simulink library "MMC_Lib"  (R2023b)
settings: Solver=VariableStepAuto  StartTime=0.0  StopTime=10.0  RelTol=1e-3
undefined symbols (not defined in the file): C_PM, D_R, D_Rs, DiscIntNeverNeededParam, Discrete, Nb_PM, spsDiodeModel, Ts_Power
libraries: simulink x23, simulink_extras x1, $bdroot x1
settings Model: Creator=rober  LastModifiedBy=rober

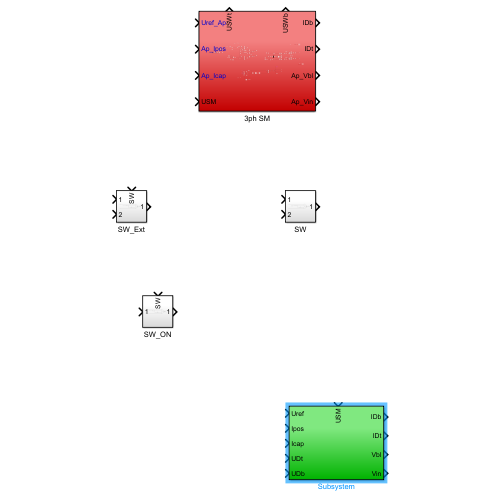
[thumbnail: Simulink's stored preview of the top-level diagram]
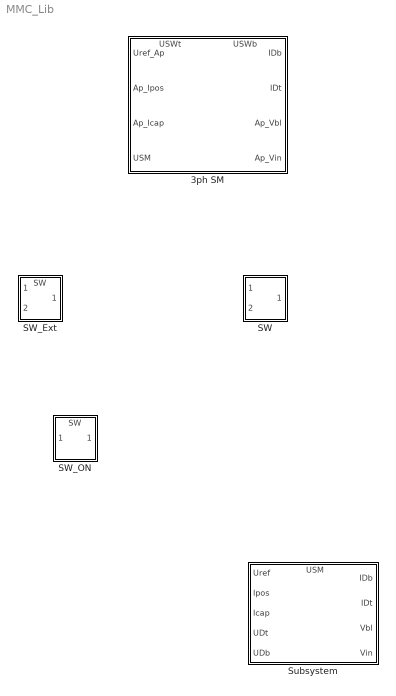
== system MMC_Lib ==
  3ph SM : Subsystem
      settings: PortSchema="{\"entries\":[{\"content\":{\"sides\":[{\"content\":{\"connectorIds\":[\"In1\",\"In2\",\"In3\",\"In4\"]},\"type\":\"ConnectorPlacement.EquallySpacedRectSide\",\"uuid\":\"e8c5836a-6fd4-401e-94d8-c7848e2937c8\"},{\"content\":{\"connectorIds\":[\"Out1\",\"Out2\",\"Out3\",\"Out4\"],\"side\":\"RIGHT\"},\"type\":\"ConnectorPlacement.EquallySpacedRectSide\",\"uuid\":\"9a1f81e7-802a-4d89-b611-499076d5a1a3\"},{\"content\":{\"connectorIds\":[\"Out5\",\"Out6\"],\"side\":\"TOP\"},\"type\":\"ConnectorPlacement.EquallySpacedRectSide\",\"uuid\":\"c5bcecc8-9b4b-4040-ad1a-25d769dc4514\"}]},\"type\":\"ConnectorPlacement.EquallySpacedConnector\",\"uuid\":\"eb5ff5d9-ed1d-4618-9338-8ec7700f9d1e\"}],\"packageUris\":[\"http://schema.mathworks.com/mf0/Connector/R2020b\"],\"version\":\"1.0\"}"
  SW : Subsystem
  SW_Ext : Subsystem
      settings: PortSchema="{\"entries\":[{\"content\":{\"sides\":[{\"content\":{\"connectorIds\":[\"In1\",\"In2\"]},\"type\":\"ConnectorPlacement.EquallySpacedRectSide\",\"uuid\":\"61570b56-e5d0-4812-b143-8fea08408b82\"},{\"content\":{\"connectorIds\":[\"Out1\"],\"side\":\"RIGHT\"},\"type\":\"ConnectorPlacement.EquallySpacedRectSide\",\"uuid\":\"fb1b449d-dcf0-4498-bfcd-c35d1b8d3af1\"},{\"content\":{\"connectorIds\":[\"In3\"],\"side\":\"TOP\"},\"type\":\"ConnectorPlacement.EquallySpacedRectSide\",\"uuid\":\"2091de1c-d6a0-4f6b-9728-c6eb9657220b\"}]},\"type\":\"ConnectorPlacement.EquallySpacedConnector\",\"uuid\":\"fce121a6-5cfd-4a9e-88a9-d62df4eca96b\"}],\"packageUris\":[\"http://schema.mathworks.com/mf0/Connector/R2020b\"],\"version\":\"1.0\"}"
  SW_ON : Subsystem
      settings: PortSchema="{\"entries\":[{\"content\":{\"sides\":[{\"content\":{\"connectorIds\":[\"In1\"]},\"type\":\"ConnectorPlacement.EquallySpacedRectSide\",\"uuid\":\"61570b56-e5d0-4812-b143-8fea08408b82\"},{\"content\":{\"connectorIds\":[\"Out1\"],\"side\":\"RIGHT\"},\"type\":\"ConnectorPlacement.EquallySpacedRectSide\",\"uuid\":\"fb1b449d-dcf0-4498-bfcd-c35d1b8d3af1\"},{\"content\":{\"connectorIds\":[\"In2\"],\"side\":\"TOP\"},\"type\":\"ConnectorPlacement.EquallySpacedRectSide\",\"uuid\":\"2091de1c-d6a0-4f6b-9728-c6eb9657220b\"}]},\"type\":\"ConnectorPlacement.EquallySpacedConnector\",\"uuid\":\"fce121a6-5cfd-4a9e-88a9-d62df4eca96b\"}],\"packageUris\":[\"http://schema.mathworks.com/mf0/Connector/R2020b\"],\"version\":\"1.0\"}"
  Subsystem : Subsystem
      settings: PortSchema="{\"entries\":[{\"content\":{\"sides\":[{\"content\":{\"connectorIds\":[\"In1\",\"In2\",\"In3\",\"In4\",\"In5\"]},\"type\":\"ConnectorPlacement.EquallySpacedRectSide\",\"uuid\":\"b7415a3a-059a-466d-a519-c19f63b714af\"},{\"content\":{\"connectorIds\":[\"Out1\",\"Out2\",\"Out3\",\"Out4\"],\"side\":\"RIGHT\"},\"type\":\"ConnectorPlacement.EquallySpacedRectSide\",\"uuid\":\"984beb61-c57c-4d2a-959b-3a61047ea667\"},{\"content\":{\"connectorIds\":[\"In6\"],\"side\":\"TOP\"},\"type\":\"ConnectorPlacement.EquallySpacedRectSide\",\"uuid\":\"184f05c1-6fe5-4e4c-8e83-c1431acf6740\"}]},\"type\":\"ConnectorPlacement.EquallySpacedConnector\",\"uuid\":\"ac4715c0-a7f3-4877-877b-fb86a389a1b7\"}],\"packageUris\":[\"http://schema.mathworks.com/mf0/Connector/R2020b\"],\"version\":\"1.0\"}"

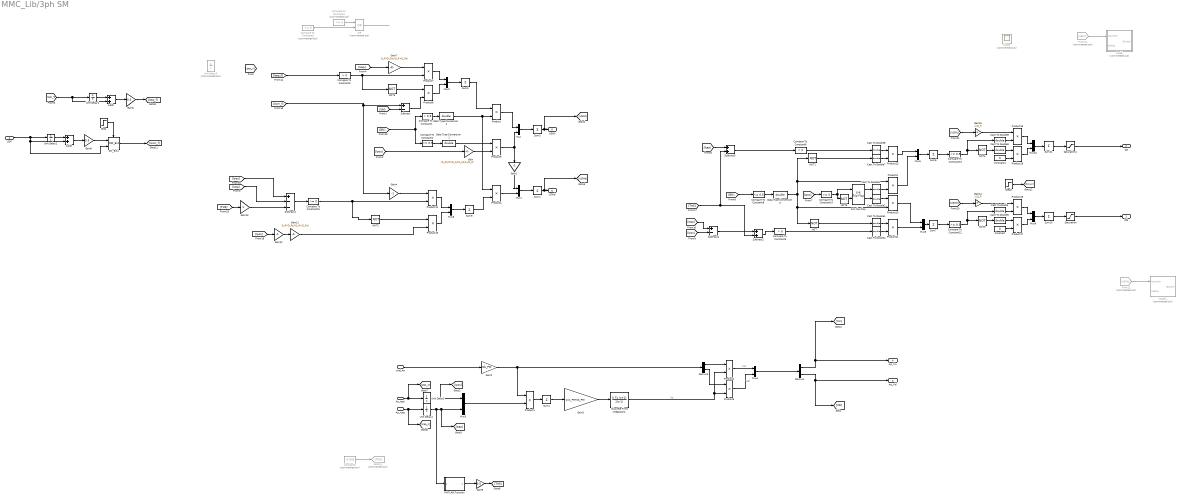
== system MMC_Lib/3ph SM ==
  Uref_Ap : Inport
  Ap_Ipos : Inport  Port=2
  Ap_Icap : Inport  Port=3
  USM : Inport  Port=4
  Add2 : Sum
  Add3 : Sum
  Cast To Double{,1..9} (10 alike) : DataTypeConversion  OutDataTypeStr=double  SaturateOnIntegerOverflow=off  RndMeth=Floor
  Compare To Constant1 : simulink/Logic and Bit Operations/Compare To Constant  relop=>  const=0.5  OutDataTypeStr=boolean
  Compare To Constant10 : simulink/Logic and Bit Operations/Compare To Constant  relop=>=  const=0  OutDataTypeStr=boolean
  Compare To Constant12 : simulink/Logic and Bit Operations/Compare To Constant  relop=>=  const=0.5  OutDataTypeStr=boolean
  Compare To Constant13 : simulink/Logic and Bit Operations/Compare To Constant  relop=>=  const=0.5  OutDataTypeStr=boolean
  Compare To Constant14 : simulink/Logic and Bit Operations/Compare To Constant  relop=>=  const=0  OutDataTypeStr=boolean
  Compare To Constant2 : simulink/Logic and Bit Operations/Compare To Constant  relop=<=  const=0.5  OutDataTypeStr=boolean
  Compare To Constant3 : simulink/Logic and Bit Operations/Compare To Constant  relop=>  const=0  OutDataTypeStr=boolean
  Compare To Constant4 : simulink/Logic and Bit Operations/Compare To Constant  Commented=on  relop=<=  const=0  OutDataTypeStr=boolean
  Compare To Constant5 : simulink/Logic and Bit Operations/Compare To Constant  Commented=on  relop=<=  const=0  OutDataTypeStr=boolean
  Compare To Constant6 : simulink/Logic and Bit Operations/Compare To Constant  relop=>  const=0  OutDataTypeStr=boolean
  Compare To Constant8 : simulink/Logic and Bit Operations/Compare To Constant  relop=<=  const=0.5  OutDataTypeStr=boolean
  Compare To Constant9 : simulink/Logic and Bit Operations/Compare To Constant  relop=>  const=0  OutDataTypeStr=boolean
  Constant : Constant  Value=0
  Constant1 : Constant  Value=0
  Constant2 : Constant  Commented=on  Value=-0.003
  Data Type Conversion1 : DataTypeConversion  OutDataTypeStr=double  SaturateOnIntegerOverflow=off  RndMeth=Floor
  Data Type Conversion2 : DataTypeConversion  OutDataTypeStr=double  SaturateOnIntegerOverflow=off  RndMeth=Floor
  Data Type Conversion3 : DataTypeConversion  OutDataTypeStr=double  SaturateOnIntegerOverflow=off  RndMeth=Floor
  Demux1 : Demux  Outputs=2
  Demux3 : Demux  Outputs=2
  Discrete-Time Integrator2 : DiscreteIntegrator  IntegratorMethod=Integration: Trapezoidal  gainval=1  SampleTime=Ts_Power  UpperSaturationLimit=5000  LowerSaturationLimit=500  ICPrevOutput=DiscIntNeverNeededParam  ICPrevScaledInput=DiscIntNeverNeededParam
  From11 : From  Commented=on  GotoTag=USWt
  From12 : From  Commented=on  GotoTag=USWb
  Gain : Gain  Gain=(D_Rs/2)*D_R/(D_Rs/2+D_R)
  Gain1 : Gain  Gain=-1
  Gain11 : Gain  Gain=D_R*D_Rs/(D_R+D_Rs)
  Gain12 : Gain  Gain=-1
  Gain13 : Gain
  Gain14 : Gain  Gain=1./D_R  SaturateOnIntegerOverflow=on  OutDataTypeStr=Inherit: Same as input  ParamDataTypeStr=Inherit: Same as input
  Gain15 : Gain  Gain=1./D_R  SaturateOnIntegerOverflow=on  OutDataTypeStr=Inherit: Same as input  ParamDataTypeStr=Inherit: Same as input
  Gain2 : Gain  Gain=Nb_PM
  Gain3 : Gain  Gain=1/(C_PM*Nb_PM)
  Gain4 : Gain  Gain=-1
  Gain5 : Gain  Gain=0.5
  Gain6 : Gain  Gain=0.5
  Gain7 : Gain  Gain=D_R*D_Rs/(D_R+D_Rs)
  Gain9 : Gain  Gain=0.5
  Goto10 : Goto  Commented=on  GotoTag=THS
  MATLAB Function : MATLAB Function  TreatAsAtomicUnit=on
  Model : Subsystem  Commented=on  AncestorBlock=spsDiodeModel/Discrete  mask(DiscreteModel){}
  Model1 : Subsystem  Commented=on  AncestorBlock=spsDiodeModel/Discrete  mask(DiscreteModel){}
  Mux{,1..6,8..10} (10 alike) : Mux  Inputs=2
  NOT{,1..6} (7 alike) : Logic  Operator=NOT  IconShape=distinctive  AllPortsSameDT=off  OutDataTypeStr=boolean
  OR : Logic  Commented=on  Operator=OR  IconShape=distinctive  AllPortsSameDT=off  OutDataTypeStr=boolean
  Product{,1..7,9..13,15..19} (18 alike) : Product
  S-R Flip-Flop : simulink_extras/Flip Flops/S-R Flip-Flop  initial_condition=0
  SW_Ext1 : $bdroot/SW_Ext  SystemSampleTime=-1  VariantActivationTime=update diagram  AllowFlexibleInterface=on  Latency=0  AutoFrameSizeCalculation=off
      settings: PortSchema="{\"entries\":[{\"content\":{\"sides\":[{\"content\":{\"connectorIds\":[\"In1\",\"In2\"]},\"type\":\"ConnectorPlacement.EquallySpacedRectSide\",\"uuid\":\"61570b56-e5d0-4812-b143-8fea08408b82\"},{\"content\":{\"connectorIds\":[\"Out1\"],\"side\":\"RIGHT\"},\"type\":\"ConnectorPlacement.EquallySpacedRectSide\",\"uuid\":\"fb1b449d-dcf0-4498-bfcd-c35d1b8d3af1\"},{\"content\":{\"connectorIds\":[\"In3\"],\"side\":\"TOP\"},\"type\":\"ConnectorPlacement.EquallySpacedRectSide\",\"uuid\":\"2091de1c-d6a0-4f6b-9728-c6eb9657220b\"}]},\"type\":\"ConnectorPlacement.EquallySpacedConnector\",\"uuid\":\"fce121a6-5cfd-4a9e-88a9-d62df4eca96b\"}],\"packageUris\":[\"http://schema.mathworks.com/mf0/Connector/R2020b\"],\"version\":\"1.0\"}"
  Saturation : Saturate  UpperLimit=inf  LowerLimit=0
  Saturation1 : Saturate  UpperLimit=inf  LowerLimit=0
  Scope : Scope  Commented=on
  Step : Step  Time=0  Before=1  After=0  SampleTime=Ts_Power
  Step2 : Step  Time=0.01  SampleTime=Ts_Power
  Subtract : Sum  Inputs=+-
  Subtract1 : Sum  Inputs=+-
  Subtract2 : Sum
  Subtract3 : Sum
  Subtract4 : Sum  Inputs=+--
  Sum{1,3..7,9..11} (9 alike) : Sum  Inputs=1  InputSameDT=on  SaturateOnIntegerOverflow=on  OutDataTypeStr=Inherit: Same as first input
  Unit Delay{1..4} (4 alike) : UnitDelay  SampleTime=Ts_Power  HasFrameUpgradeWarning=on
  Unit Delay5 : UnitDelay  Commented=on  SampleTime=Ts_Power  HasFrameUpgradeWarning=on
  IDb : Outport
  IDt : Outport  Port=2
  Ap_Vbl : Outport  Port=3
  Ap_Vin : Outport  Port=4
  USWt : Outport  Port=5
  USWb : Outport  Port=6
  wires:
  Mux3/1 -> Product1/2
  Product1/1 -> Sum1/1
  Sum1/1 -> Gain3/1
  Discrete-Time Integrator2/1 -> Product5/2, Product2/2  "Vc"
  Uref_Ap/1 -> Gain2/1
  Demux3/2 -> Product5/1
  Gain3/1 -> Discrete-Time Integrator2/1
  Gain2/1 -> Demux3/1, Product1/1
  Demux3/1 -> Product2/1
  Mux4/1 -> Demux1/1
  Product2/1 -> Mux4/1  "Vin"
  Product5/1 -> Mux4/2  "Vbl"
  Compare To Constant1/1 -> Data Type Conversion2/1
  [Blk] -> Compare To Constant1/1, Compare To Constant2/1
  [Vbl] -> Subtract/2
  Product/1 -> Mux/1
  Unit Delay4/1 -> MATLAB Function/1(u), [Icap], Mux3/2
  Mux/1 -> Sum3/1
  Sum3/1 -> [USWt], USWt/1
  Unit Delay3/1 -> [Ipos], Mux3/1
  Compare To Constant2/1 -> Data Type Conversion1/1
  Data Type Conversion1/1 -> Product3/1
  Data Type Conversion2/1 -> Product4/1, Product/2
  Product3/1 -> Mux/2, Gain1/1
  Subtract/1 -> Product6/2
  Gain/1 -> Product3/2
  Sum4/1 -> [USWb], USWb/1
  Mux1/1 -> Sum4/1
  Gain1/1 -> Mux1/1
  Sum5/1 -> Product/1
  Compare To Constant3/1 -> NOT5/1, Product7/2
  Gain7/1 -> Product7/1
  Mux2/1 -> Sum5/1
  Product6/1 -> Mux2/2
  Product7/1 -> Mux2/1
  [Ipos] -> Gain/1
  [Icap] -> Gain7/1
  [Icap_f] -> Compare To Constant3/1
  Mux5/1 -> Sum6/1
  Data Type Conversion3/1 -> NOT/1, Product10/2, NOT1/1, Product9/1
  [Blk] -> Compare To Constant8/1
  Compare To Constant8/1 -> Data Type Conversion3/1
  Mux6/1 -> Sum7/1
  [Ipos] -> Compare To Constant14/1
  Compare To Constant14/1 -> S-R Flip-Flop/1, NOT6/1
  NOT6/1 -> S-R Flip-Flop/2
  S-R Flip-Flop/2 -> Cast To Double2/1
  S-R Flip-Flop/1 -> Cast To Double3/1
  Cast To Double3/1 -> Product9/2
  Cast To Double2/1 -> Product10/1
  Product9/1 -> Mux5/2
  Product10/1 -> Mux6/1
  [Icap] -> Subtract1/1
  [Ipos] -> Subtract1/2
  Compare To Constant9/1 -> Cast To Double4/1
  Subtract1/1 -> Subtract2/1
  NOT/1 -> Cast To Double1/1
  Cast To Double1/1 -> Product11/1
  Cast To Double4/1 -> Product11/2
  Subtract2/1 -> Compare To Constant9/1
  Subtract3/1 -> Compare To Constant6/1
  [Icap] -> Subtract3/1
  MATLAB Function/1(y) -> Gain9/1
  [THS] -> Subtract2/2, Subtract3/2
  Product11/1 -> Mux6/2
  Compare To Constant6/1 -> Cast To Double8/1
  Product13/1 -> Mux5/1
  NOT1/1 -> Cast To Double7/1
  Cast To Double7/1 -> Product13/2
  Cast To Double8/1 -> Product13/1
  Gain4/1 -> Product12/1
  Product4/1 -> Mux1/2
  Subtract4/1 -> Compare To Constant10/1
  Gain9/1 -> [THS]
  [THS] -> Gain13/1
  Product12/1 -> Mux8/1
  Sum9/1 -> Product4/2
  Mux8/1 -> Sum9/1
  Product15/1 -> Mux8/2
  NOT2/1 -> Product15/1
  [Ipos] -> Gain12/1
  Gain11/1 -> Product15/2
  Gain12/1 -> Gain11/1
  Gain13/1 -> Subtract4/3
  Compare To Constant10/1 -> NOT2/1, Product12/2
  [Icap] -> Subtract4/2
  [Ipos] -> Subtract4/1
  Compare To Constant12/1 -> Cast To Double/1, NOT3/1
  [USWb] -> Gain14/1
  NOT3/1 -> Cast To Double5/1
  Mux9/1 -> Sum10/1
  Product16/1 -> Mux9/1
  Product17/1 -> Mux9/2
  Sum10/1 -> Saturation/1
  Cast To Double/1 -> Product16/2
  Cast To Double5/1 -> Product17/1
  Constant/1 -> Product17/2
  Gain14/1 -> Product16/1
  From12/1 -> Model1/1(Uswitch)
  ? -> Model1/2(status)
  Sum7/1 -> Compare To Constant12/1
  Compare To Constant13/1 -> Cast To Double6/1, NOT4/1
  NOT4/1 -> Cast To Double9/1
  Mux10/1 -> Sum11/1
  Constant1/1 -> Product19/2
  Product19/1 -> Mux10/2
  Product18/1 -> Mux10/1
  Cast To Double9/1 -> Product19/1
  [USWt] -> Gain15/1
  Gain15/1 -> Product18/1
  Cast To Double6/1 -> Product18/2
  Sum11/1 -> Saturation1/1
  From11/1 -> Model/1(Uswitch)
  ? -> Model/2(status)
  Sum6/1 -> Compare To Constant13/1
  [Usm_f] -> Gain4/1, Subtract/1
  OR/1 -> ?
  Compare To Constant5/1 -> OR/2
  ? -> Compare To Constant4/1
  Compare To Constant4/1 -> OR/1
  NOT5/1 -> Product6/1
  Ap_Ipos/1 -> [Ipos_n], Unit Delay3/1
  Ap_Icap/1 -> [Icap_n], Unit Delay4/1
  [Icap_n] -> Unit Delay1/1, Add2/2
  Unit Delay1/1 -> Add2/1
  Add2/1 -> Gain5/1
  Gain5/1 -> [Icap_f]
  Constant2/1 -> Goto10/1
  Unit Delay2/1 -> Add3/1
  Add3/1 -> Gain6/1
  USM/1 -> Unit Delay2/1, SW_Ext1/2, Add3/2
  Gain6/1 -> SW_Ext1/1
  SW_Ext1/1 -> [Usm_f]
  Step/1 -> SW_Ext1/3
  Demux1/1 -> Ap_Vin/1, [Vin]
  Demux1/2 -> Ap_Vbl/1, [Vbl]
  Saturation/1 -> IDb/1
  Saturation1/1 -> IDt/1
  Step2/1 -> [SW_on]

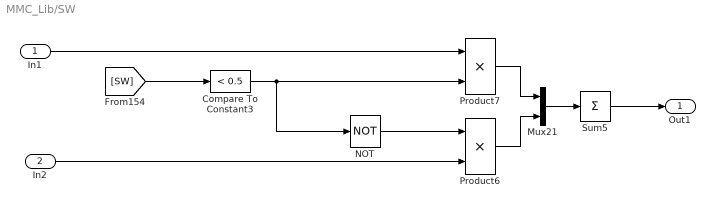
== system MMC_Lib/SW ==
  In1 : Inport
  In2 : Inport  Port=2
  Compare To Constant3 : simulink/Logic and Bit Operations/Compare To Constant  relop=<  const=0.5  OutDataTypeStr=boolean
  Mux21 : Mux  Inputs=2
  NOT : Logic  Operator=NOT  IconShape=distinctive  AllPortsSameDT=off  OutDataTypeStr=boolean
  Product6 : Product
  Product7 : Product
  Sum5 : Sum  Inputs=1  InputSameDT=on  SaturateOnIntegerOverflow=on  OutDataTypeStr=Inherit: Same as first input
  Out1 : Outport
  wires:
  In2/1 -> Product6/2
  Compare To Constant3/1 -> NOT/1, Product7/2
  Product7/1 -> Mux21/1
  [SW] -> Compare To Constant3/1
  In1/1 -> Product7/1
  NOT/1 -> Product6/1
  Product6/1 -> Mux21/2
  Mux21/1 -> Sum5/1
  Sum5/1 -> Out1/1

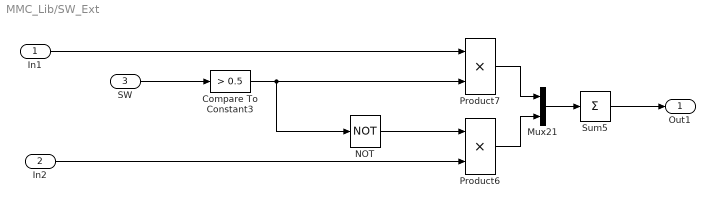
== system MMC_Lib/SW_Ext ==
  In1 : Inport
  In2 : Inport  Port=2
  SW : Inport  Port=3
  Compare To Constant3 : simulink/Logic and Bit Operations/Compare To Constant  relop=>  const=0.5  OutDataTypeStr=boolean
  Mux21 : Mux  Inputs=2
  NOT : Logic  Operator=NOT  IconShape=distinctive  AllPortsSameDT=off  OutDataTypeStr=boolean
  Product6 : Product
  Product7 : Product
  Sum5 : Sum  Inputs=1  InputSameDT=on  SaturateOnIntegerOverflow=on  OutDataTypeStr=Inherit: Same as first input
  Out1 : Outport
  wires:
  In2/1 -> Product6/2
  Compare To Constant3/1 -> NOT/1, Product7/2
  Product7/1 -> Mux21/1
  SW/1 -> Compare To Constant3/1
  In1/1 -> Product7/1
  NOT/1 -> Product6/1
  Product6/1 -> Mux21/2
  Mux21/1 -> Sum5/1
  Sum5/1 -> Out1/1

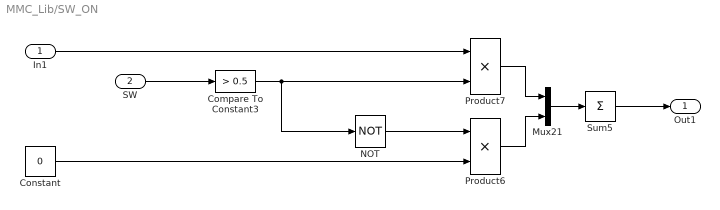
== system MMC_Lib/SW_ON ==
  In1 : Inport
  SW : Inport  Port=2
  Compare To Constant3 : simulink/Logic and Bit Operations/Compare To Constant  relop=>  const=0.5  OutDataTypeStr=boolean
  Constant : Constant  Value=0
  Mux21 : Mux  Inputs=2
  NOT : Logic  Operator=NOT  IconShape=distinctive  AllPortsSameDT=off  OutDataTypeStr=boolean
  Product6 : Product
  Product7 : Product
  Sum5 : Sum  Inputs=1  InputSameDT=on  SaturateOnIntegerOverflow=on  OutDataTypeStr=Inherit: Same as first input
  Out1 : Outport
  wires:
  Sum5/1 -> Out1/1
  Mux21/1 -> Sum5/1
  Product6/1 -> Mux21/2
  NOT/1 -> Product6/1
  In1/1 -> Product7/1
  SW/1 -> Compare To Constant3/1
  Product7/1 -> Mux21/1
  Compare To Constant3/1 -> Product7/2, NOT/1
  Constant/1 -> Product6/2

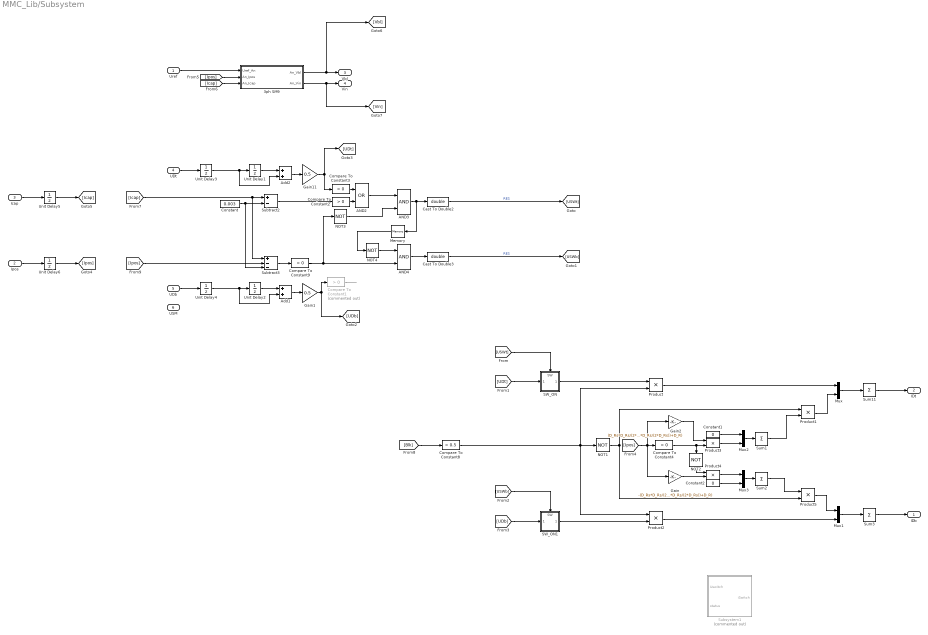
== system MMC_Lib/Subsystem ==
  Uref : Inport
  Ipos : Inport  Port=2
  Icap : Inport  Port=3
  UDt : Inport  Port=4
  UDb : Inport  Port=5
  USM : Inport  Port=6
  3ph SM9 : Subsystem
  AND2 : Logic  Operator=OR  IconShape=distinctive  AllPortsSameDT=off  OutDataTypeStr=boolean
  AND3 : Logic  IconShape=distinctive  AllPortsSameDT=off  OutDataTypeStr=boolean
  AND4 : Logic  IconShape=distinctive  AllPortsSameDT=off  OutDataTypeStr=boolean
  Add1 : Sum
  Add2 : Sum
  Cast To Double2 : DataTypeConversion  OutDataTypeStr=double  SaturateOnIntegerOverflow=off  RndMeth=Floor
  Cast To Double3 : DataTypeConversion  OutDataTypeStr=double  SaturateOnIntegerOverflow=off  RndMeth=Floor
  Compare To Constant1 : simulink/Logic and Bit Operations/Compare To Constant  Commented=on  relop=>  const=0  OutDataTypeStr=boolean
  Compare To Constant{2..4,9} (4 alike) : simulink/Logic and Bit Operations/Compare To Constant  relop=>  const=0  OutDataTypeStr=boolean
  Compare To Constant8 : simulink/Logic and Bit Operations/Compare To Constant  relop=>  const=0.5  OutDataTypeStr=boolean
  Constant : Constant  Value=0.003
  Constant1 : Constant  Value=0
  Constant2 : Constant  Value=0
  Gain : Gain  Gain=-(D_Rs*D_Rs/(2*D_Rs))/((D_Rs*D_Rs/(2*D_Rs))+D_R)
  Gain1 : Gain  Gain=0.5
  Gain11 : Gain  Gain=0.5
  Gain2 : Gain  Gain=(D_Rs*D_Rs/(2*D_Rs))/((D_Rs*D_Rs/(2*D_Rs))+D_R)
  Memory : Memory
  Mux{,1..3} (4 alike) : Mux  Inputs=2
  NOT{1..4} (4 alike) : Logic  Operator=NOT  IconShape=distinctive  AllPortsSameDT=off  OutDataTypeStr=boolean
  Product{,1..5} (6 alike) : Product
  SW_ON : Subsystem
      settings: PortSchema="{\"entries\":[{\"content\":{\"sides\":[{\"content\":{\"connectorIds\":[\"In1\"]},\"type\":\"ConnectorPlacement.EquallySpacedRectSide\",\"uuid\":\"61570b56-e5d0-4812-b143-8fea08408b82\"},{\"content\":{\"connectorIds\":[\"Out1\"],\"side\":\"RIGHT\"},\"type\":\"ConnectorPlacement.EquallySpacedRectSide\",\"uuid\":\"fb1b449d-dcf0-4498-bfcd-c35d1b8d3af1\"},{\"content\":{\"connectorIds\":[\"In2\"],\"side\":\"TOP\"},\"type\":\"ConnectorPlacement.EquallySpacedRectSide\",\"uuid\":\"2091de1c-d6a0-4f6b-9728-c6eb9657220b\"}]},\"type\":\"ConnectorPlacement.EquallySpacedConnector\",\"uuid\":\"fce121a6-5cfd-4a9e-88a9-d62df4eca96b\"}],\"packageUris\":[\"http://schema.mathworks.com/mf0/Connector/R2020b\"],\"version\":\"1.0\"}"
  SW_ON1 : Subsystem
      settings: PortSchema="{\"entries\":[{\"content\":{\"sides\":[{\"content\":{\"connectorIds\":[\"In1\"]},\"type\":\"ConnectorPlacement.EquallySpacedRectSide\",\"uuid\":\"61570b56-e5d0-4812-b143-8fea08408b82\"},{\"content\":{\"connectorIds\":[\"Out1\"],\"side\":\"RIGHT\"},\"type\":\"ConnectorPlacement.EquallySpacedRectSide\",\"uuid\":\"fb1b449d-dcf0-4498-bfcd-c35d1b8d3af1\"},{\"content\":{\"connectorIds\":[\"In2\"],\"side\":\"TOP\"},\"type\":\"ConnectorPlacement.EquallySpacedRectSide\",\"uuid\":\"2091de1c-d6a0-4f6b-9728-c6eb9657220b\"}]},\"type\":\"ConnectorPlacement.EquallySpacedConnector\",\"uuid\":\"fce121a6-5cfd-4a9e-88a9-d62df4eca96b\"}],\"packageUris\":[\"http://schema.mathworks.com/mf0/Connector/R2020b\"],\"version\":\"1.0\"}"
  Subsystem1 : Subsystem  Commented=on
  Subtract2 : Sum  Inputs=+-
  Subtract3 : Sum  Inputs=+--
  Sum{1..3,11} (4 alike) : Sum  Inputs=1  InputSameDT=on  SaturateOnIntegerOverflow=on  OutDataTypeStr=Inherit: Same as first input
  Unit Delay{1..6} (6 alike) : UnitDelay  SampleTime=Ts_Power  HasFrameUpgradeWarning=on
  IDb : Outport
  IDt : Outport  Port=2
  Vbl : Outport  Port=3
  Vin : Outport  Port=4
  wires:
  UDt/1 -> Unit Delay3/1
  Constant/1 -> Subtract3/3, Subtract2/2
  Ipos/1 -> Unit Delay6/1
  NOT4/1 -> AND4/1
  AND2/1 -> AND3/1
  NOT3/1 -> AND3/2
  Gain11/1 -> [UDt], Compare To Constant3/1
  Compare To Constant3/1 -> AND2/1
  Unit Delay1/1 -> Add2/1
  Add2/1 -> Gain11/1
  Cast To Double2/1 -> [USWt]  "RES"
  Subtract3/1 -> Compare To Constant9/1
  Subtract2/1 -> Compare To Constant2/1
  AND3/1 -> Cast To Double2/1, Memory/1
  Compare To Constant2/1 -> AND2/2
  Cast To Double3/1 -> [USWb]  "RES"
  AND4/1 -> Cast To Double3/1
  Icap/1 -> Unit Delay5/1
  Memory/1 -> NOT4/1
  Compare To Constant9/1 -> AND4/2, NOT3/1
  UDb/1 -> Unit Delay4/1
  Unit Delay2/1 -> Add1/1
  Add1/1 -> Gain1/1
  Gain1/1 -> [UDb], Compare To Constant1/1
  Compare To Constant1/1 -> ?
  [USWt] -> SW_ON/2(SW)
  [UDt] -> SW_ON/1(In1)
  [UDb] -> SW_ON1/1(In1)
  [USWb] -> SW_ON1/2(SW)
  [Blk] -> Compare To Constant8/1
  Compare To Constant8/1 -> Product/2, NOT1/1, Product2/1
  SW_ON/1(Out1) -> Product/1
  Product/1 -> Mux/1
  NOT1/1 -> Product1/1, Product5/2
  Product1/1 -> Mux/2
  SW_ON1/1(Out1) -> Product2/2
  Product2/1 -> Mux1/2
  Mux1/1 -> Sum3/1
  Sum11/1 -> IDt/1
  Mux/1 -> Sum11/1
  Mux2/1 -> Sum1/1
  Product3/1 -> Mux2/2
  Sum1/1 -> Product1/2
  [Ipos] -> Gain2/1, Compare To Constant4/1, Gain/1
  Compare To Constant4/1 -> NOT2/1, Product3/2
  Product4/1 -> Mux3/1
  Mux3/1 -> Sum2/1
  Sum2/1 -> Product5/1
  Constant2/1 -> Mux3/2
  Product5/1 -> Mux1/1
  NOT2/1 -> Product4/1
  Gain/1 -> Product4/2
  Sum3/1 -> IDb/1
  Gain2/1 -> Product3/1
  Constant1/1 -> Mux2/1
  [Ipos] -> 3ph SM9/2(An_Ipos)
  [Icap] -> 3ph SM9/3(An_Icap)
  Uref/1 -> 3ph SM9/1(Uref_An)
  3ph SM9/1(An_Vbl) -> [Vbl], Vbl/1
  3ph SM9/2(An_Vin) -> [Vin], Vin/1
  [Icap] -> Subtract3/1, Subtract2/1
  Unit Delay5/1 -> [Icap]
  [Ipos] -> Subtract3/2
  Unit Delay6/1 -> [Ipos]
  Unit Delay3/1 -> Add2/2, Unit Delay1/1
  Unit Delay4/1 -> Add1/2, Unit Delay2/1

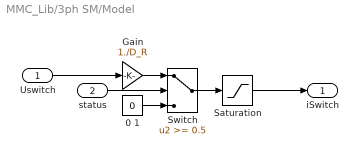
== system MMC_Lib/3ph SM/Model ==
  Uswitch : Inport
  status : Inport  Port=2
  0 1 : Constant  Value=0
  Gain : Gain  Gain=1./D_R  SaturateOnIntegerOverflow=on  OutDataTypeStr=Inherit: Same as input  ParamDataTypeStr=Inherit: Same as input
  Saturation : Saturate  UpperLimit=inf  LowerLimit=0
  Switch : Switch  Threshold=0.5  SaturateOnIntegerOverflow=off
  iSwitch : Outport
  wires:
  Uswitch/1 -> Gain/1
  Gain/1 -> Switch/1
  0 1/1 -> Switch/3
  Switch/1 -> Saturation/1
  Saturation/1 -> iSwitch/1
  status/1 -> Switch/2

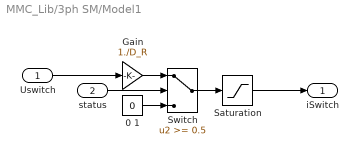
== system MMC_Lib/3ph SM/Model1 ==
  Uswitch : Inport
  status : Inport  Port=2
  0 1 : Constant  Value=0
  Gain : Gain  Gain=1./D_R  SaturateOnIntegerOverflow=on  OutDataTypeStr=Inherit: Same as input  ParamDataTypeStr=Inherit: Same as input
  Saturation : Saturate  UpperLimit=inf  LowerLimit=0
  Switch : Switch  Threshold=0.5  SaturateOnIntegerOverflow=off
  iSwitch : Outport
  wires:
  Uswitch/1 -> Gain/1
  Gain/1 -> Switch/1
  0 1/1 -> Switch/3
  Switch/1 -> Saturation/1
  Saturation/1 -> iSwitch/1
  status/1 -> Switch/2

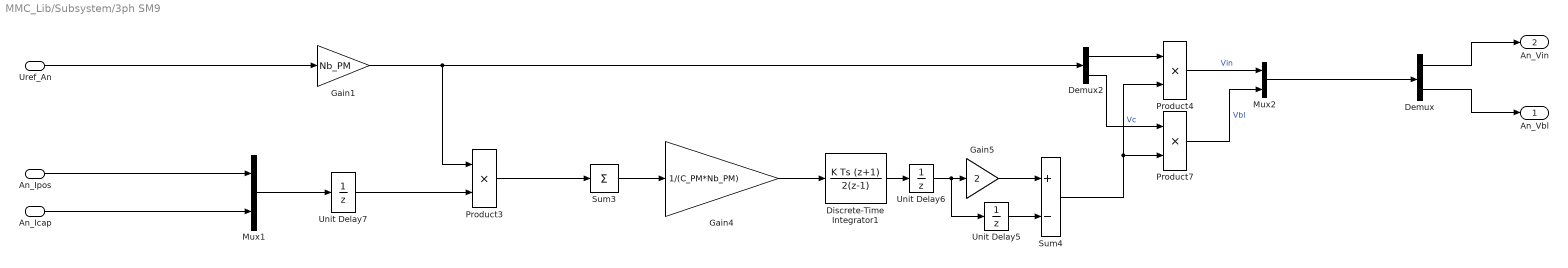
== system MMC_Lib/Subsystem/3ph SM9 ==
  Uref_An : Inport
  An_Ipos : Inport  Port=2
  An_Icap : Inport  Port=3
  Demux : Demux  Outputs=2
  Demux2 : Demux  Outputs=2
  Discrete-Time Integrator1 : DiscreteIntegrator  IntegratorMethod=Integration: Trapezoidal  gainval=1  SampleTime=Ts_Power  UpperSaturationLimit=5000  LowerSaturationLimit=500  ICPrevOutput=DiscIntNeverNeededParam  ICPrevScaledInput=DiscIntNeverNeededParam
  Gain1 : Gain  Gain=Nb_PM
  Gain4 : Gain  Gain=1/(C_PM*Nb_PM)
  Gain5 : Gain  Gain=2
  Mux1 : Mux  Inputs=2
  Mux2 : Mux  Inputs=2
  Product3 : Product
  Product4 : Product
  Product7 : Product
  Sum3 : Sum  Inputs=1  InputSameDT=on  SaturateOnIntegerOverflow=on  OutDataTypeStr=Inherit: Same as first input
  Sum4 : Sum  Inputs=+-  InputSameDT=on  SaturateOnIntegerOverflow=on  OutDataTypeStr=Inherit: Same as first input
  Unit Delay5 : UnitDelay  SampleTime=Ts_Power  HasFrameUpgradeWarning=on
  Unit Delay6 : UnitDelay  SampleTime=Ts_Power  HasFrameUpgradeWarning=on
  Unit Delay7 : UnitDelay  SampleTime=Ts_Power  HasFrameUpgradeWarning=on
  An_Vbl : Outport
  An_Vin : Outport  Port=2
  wires:
  Gain5/1 -> Sum4/1
  Gain1/1 -> Demux2/1, Product3/1
  Mux2/1 -> Demux/1
  Demux/1 -> An_Vin/1
  Uref_An/1 -> Gain1/1
  Gain4/1 -> Discrete-Time Integrator1/1
  Mux1/1 -> Unit Delay7/1
  Demux2/2 -> Product7/1
  Unit Delay6/1 -> Gain5/1, Unit Delay5/1
  An_Icap/1 -> Mux1/2
  Demux2/1 -> Product4/1
  Discrete-Time Integrator1/1 -> Unit Delay6/1
  Sum4/1 -> Product7/2, Product4/2  "Vc"
  Unit Delay5/1 -> Sum4/2
  Sum3/1 -> Gain4/1
  Product3/1 -> Sum3/1
  Product4/1 -> Mux2/1  "Vin"
  Demux/2 -> An_Vbl/1
  Product7/1 -> Mux2/2  "Vbl"
  Unit Delay7/1 -> Product3/2
  An_Ipos/1 -> Mux1/1

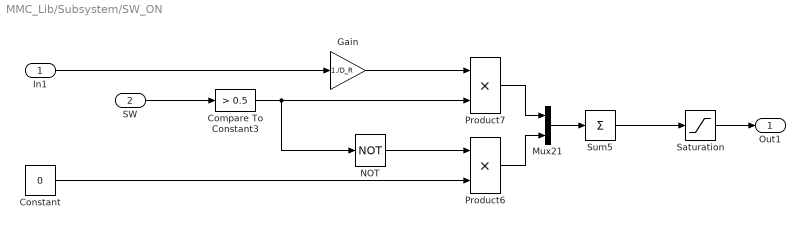
== system MMC_Lib/Subsystem/SW_ON ==
  In1 : Inport
  SW : Inport  Port=2
  Compare To Constant3 : simulink/Logic and Bit Operations/Compare To Constant  relop=>  const=0.5  OutDataTypeStr=boolean
  Constant : Constant  Value=0
  Gain : Gain  Gain=1./D_R  SaturateOnIntegerOverflow=on  OutDataTypeStr=Inherit: Same as input  ParamDataTypeStr=Inherit: Same as input
  Mux21 : Mux  Inputs=2
  NOT : Logic  Operator=NOT  IconShape=distinctive  AllPortsSameDT=off  OutDataTypeStr=boolean
  Product6 : Product
  Product7 : Product
  Saturation : Saturate  UpperLimit=inf  LowerLimit=0
  Sum5 : Sum  Inputs=1  InputSameDT=on  SaturateOnIntegerOverflow=on  OutDataTypeStr=Inherit: Same as first input
  Out1 : Outport
  wires:
  Sum5/1 -> Saturation/1
  Mux21/1 -> Sum5/1
  Product6/1 -> Mux21/2
  NOT/1 -> Product6/1
  In1/1 -> Gain/1
  SW/1 -> Compare To Constant3/1
  Product7/1 -> Mux21/1
  Compare To Constant3/1 -> Product7/2, NOT/1
  Constant/1 -> Product6/2
  Gain/1 -> Product7/1
  Saturation/1 -> Out1/1

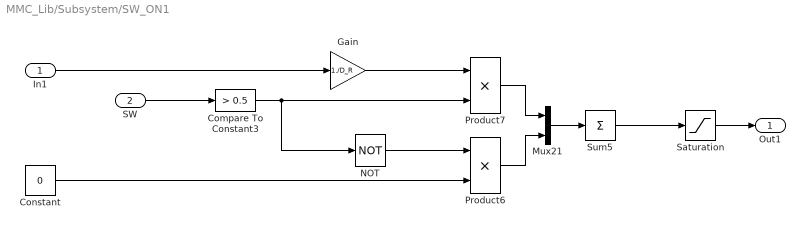
== system MMC_Lib/Subsystem/SW_ON1 ==
  In1 : Inport
  SW : Inport  Port=2
  Compare To Constant3 : simulink/Logic and Bit Operations/Compare To Constant  relop=>  const=0.5  OutDataTypeStr=boolean
  Constant : Constant  Value=0
  Gain : Gain  Gain=1./D_R  SaturateOnIntegerOverflow=on  OutDataTypeStr=Inherit: Same as input  ParamDataTypeStr=Inherit: Same as input
  Mux21 : Mux  Inputs=2
  NOT : Logic  Operator=NOT  IconShape=distinctive  AllPortsSameDT=off  OutDataTypeStr=boolean
  Product6 : Product
  Product7 : Product
  Saturation : Saturate  UpperLimit=inf  LowerLimit=0
  Sum5 : Sum  Inputs=1  InputSameDT=on  SaturateOnIntegerOverflow=on  OutDataTypeStr=Inherit: Same as first input
  Out1 : Outport
  wires:
  Sum5/1 -> Saturation/1
  Mux21/1 -> Sum5/1
  Product6/1 -> Mux21/2
  NOT/1 -> Product6/1
  In1/1 -> Gain/1
  SW/1 -> Compare To Constant3/1
  Product7/1 -> Mux21/1
  Compare To Constant3/1 -> Product7/2, NOT/1
  Constant/1 -> Product6/2
  Gain/1 -> Product7/1
  Saturation/1 -> Out1/1

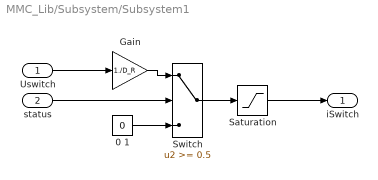
== system MMC_Lib/Subsystem/Subsystem1 ==
  Uswitch : Inport
  status : Inport  Port=2
  0 1 : Constant  Value=0
  Gain : Gain  Gain=1./D_R  SaturateOnIntegerOverflow=on  OutDataTypeStr=Inherit: Same as input  ParamDataTypeStr=Inherit: Same as input
  Saturation : Saturate  UpperLimit=inf  LowerLimit=0
  Switch : Switch  Threshold=0.5  SaturateOnIntegerOverflow=off
  iSwitch : Outport
  wires:
  status/1 -> Switch/2
  0 1/1 -> Switch/3
  Gain/1 -> Switch/1
  Switch/1 -> Saturation/1
  Saturation/1 -> iSwitch/1
  Uswitch/1 -> Gain/1

== matlab function MMC_Lib/3ph SM/MATLAB Function ==
  data: u input; y output
function y = fcn(u)

persistent min;

if(isempty(min)) min =  -0.001; end


if(u < min) min = u; end

y = min;

end
